simulink model "Controller3_PID"  (R2021b)
settings: Solver=VariableStepAuto  StartTime=0.0  StopTime=10.0  RelTol=1e-3
libraries: simulink_extras x2
settings Model: Creator=david  LastModifiedBy=david

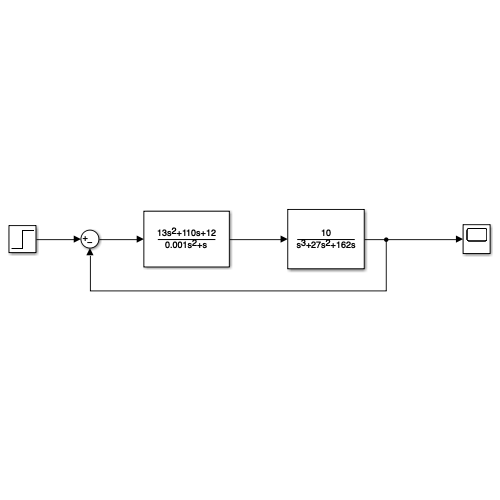
[thumbnail: Simulink's stored preview of the top-level diagram]
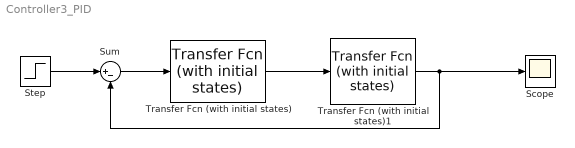
== system Controller3_PID ==
  Scope : Scope
  Step : Step  Time=0  SampleTime=0
  Sum : Sum  Inputs=|+-
  Transfer Fcn (with initial states) : simulink_extras/Additional Linear/Transfer Fcn (with initial states)  N=[13 110 12]  D=[.001 1 0]  X0=0
  Transfer Fcn (with initial states)1 : simulink_extras/Additional Linear/Transfer Fcn (with initial states)  N=[10]  D="[1  27 162 0]"  X0=0
  wires:
  Sum/1 -> Transfer Fcn (with initial states)/1
  Step/1 -> Sum/1
  Transfer Fcn (with initial states)1/1 -> Scope/1, Sum/2
  Transfer Fcn (with initial states)/1 -> Transfer Fcn (with initial states)1/1
